simulink model "UDPSendBlockReceiveBlock"  (R2017b)
settings: Solver=FixedStepDiscrete  StartTime=0.0  StopTime=10.0  FixedStep=1e-3  RelTol=1e-3
libraries: mbed_lib x3, mbed_ethernet_udp x3, mbed_ethernet x1
settings Model: Creator=oh  LastModifiedBy=oh
settings OptimizationCC: DefaultParameterBehavior=Inlined
settings DebuggingCC: ParameterTunabilityLossMsg=error
settings HardwareCC: ProdBitPerPointer=32  ProdBitPerSizeT=32  ProdBitPerPtrDiffT=32  ProdLargestAtomicInteger=Long  ProdLargestAtomicFloat=Double  ProdWordSize=32  ProdHWDeviceType=ARM Compatible->ARM Cortex
settings SFSimCC: MATLABDynamicMemAlloc=off
settings RTWCC: SystemTargetFile=mbed.tlc  TemplateMakefile=mbed.tmf  Description=MbedTarget (Embedded Target for Embedded Coder)  IncludeHyperlinkInReport=on  TargetLang=C++
settings CodeAppCC: ForceParamTrailComments=on  IgnoreCustomStorageClasses=off  OperatorAnnotations=on  SimulinkDataObjDesc=on  SFDataObjDesc=on  MATLABFcnDesc=on  InsertBlockDesc=on  StateflowObjectComments=on  MATLABSourceComments=on
settings STFCustomTargetCC: TargetLibSuffix=.a  TargetLangStandard=C++03 (ISO)  GenerateSampleERTMain=on  CombineOutputUpdateFcns=on  ERTCustomFileBanners=on  SupportContinuousTime=off  SupportNonInlinedSFcns=off  RemoveResetFunc=on  MATLABClassNameForMDSCustomization=Simulink.SoftwareTarget.ERTCustomization  ModelStepFunctionPrototypeControlCompliant=on  GRTInterface=off  SystemTargetFile=mbed.tlc
settings ERTTargetCC: TargetLangStandard=C++03 (ISO)  MultiwordLength=2048  GenerateSampleERTMain=on  ParMdlRefBuildCompliant=off  CompOptLevelCompliant=off  ConcurrentExecutionCompliant=off  CPPClassGenCompliant=off  UseToolchainInfoCompliant=off  InlinedParameterPlacement=NonHierarchical  ERTCustomFileTemplate=mbed_file_process.tlc

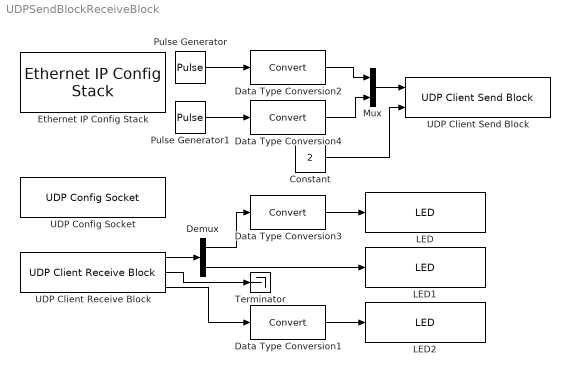
== system UDPSendBlockReceiveBlock ==
  Constant : Constant  Value=2  OutDataTypeStr=uint32
  Data Type Conversion{1..4} (4 alike) : DataTypeConversion
  Demux : Demux  Outputs=2
  Ethernet IP Config Stack : mbed_ethernet/Ethernet IP Config Stack  Priority=0  sDHCP=off  DHCP=0  ip_addr=192.168.178.200  sub_mask=255.255.255.0  gateway=0.0.0.0  SerialDebugInfo=on
      settings: SourceProductName=Mbed Target
  LED : mbed_lib/GPIO/LED  nLED=1  SampleTime=-1
      settings: SourceProductName=Mbed Target
  LED1 : mbed_lib/GPIO/LED  nLED=2  SampleTime=-1
      settings: SourceProductName=Mbed Target
  LED2 : mbed_lib/GPIO/LED  nLED=3  SampleTime=-1
      settings: SourceProductName=Mbed Target
  Mux : Mux  Inputs=2
  Pulse Generator : DiscretePulseGenerator  PulseType=Time based  PulseWidth=50
  Pulse Generator1 : DiscretePulseGenerator  PulseType=Time based  PulseWidth=50  PhaseDelay=1
  Terminator : Terminator
  UDP Client Receive Block : mbed_ethernet_udp/UDP Client Receive Block  sock_ID=1  BufferSize=2  Blocking=off  ErrorOutputport=on  SampleTime=1
      settings: SourceProductName=Mbed Target
  UDP Client Send Block : mbed_ethernet_udp/UDP Client Send Block  sock_ID=1  numData=on  SampleTime=1
      settings: SourceProductName=Mbed Target
  UDP Config Socket : mbed_ethernet_udp/UDP Config Socket  Priority=1  des_IP=192.168.178.25  des_port=10001  sock_ID=1
      settings: SourceProductName=Mbed Target
  wires:
  Demux/1 -> Data Type Conversion3/1
  Data Type Conversion1/1 -> LED2/1
  Demux/2 -> LED1/1
  Data Type Conversion3/1 -> LED/1
  UDP Client Receive Block/3 -> Data Type Conversion1/1
  Pulse Generator/1 -> Data Type Conversion2/1
  Data Type Conversion4/1 -> Mux/2
  Pulse Generator1/1 -> Data Type Conversion4/1
  Data Type Conversion2/1 -> Mux/1
  Mux/1 -> UDP Client Send Block/1
  UDP Client Receive Block/1 -> Demux/1
  Constant/1 -> UDP Client Send Block/2
  UDP Client Receive Block/2 -> Terminator/1
